simulink model "top_model"  (R2017a)
settings: Solver=ode23t  StartTime=0.0  StopTime=100  FixedStep=0.005  MaxStep=0.05  RelTol=1e-8  EnableMultiTasking=on
InitFcn:
  | load('DrivenData.mat');
  | load('vehicleParameters.mat');
undefined symbols (not defined in the file): B, C, CA, Cd, Cl, cogHeight, D, E, F, frontArea, frontBrakeBias, mass, maxBrakingTorque, maxPower, maxTorque, P, R, rearWeightDist, trackWidth, wheelBase
(part 1 of 2)
settings Model: Creator=The MathWorks, Inc.  LastModifiedBy=Jianming
settings SolverCC: MaxConsecutiveMinStep=5
settings DataIOCC: LimitDataPoints=on
settings OptimizationCC: LifeSpan=inf
settings DebuggingCC: AllowSymbolicDim=off  SFUnexpectedBacktrackingDiag=warning  SFNoUnconditionalDefaultTransitionDiag=warning  SFExecutionAtInitializationDiag=none
settings ModelReferenceCC: PropagateSignalLabelsOutOfModel=off
settings GRTTargetCC: TargetLangStandard=C89/C90 (ANSI)
settings ConfigComp: CovMetricSettings=dw  CovHtmlReporting=on  CovSaveCumulativeToWorkspaceVar=on  CovSaveSingleToWorkspaceVar=on  CovExternalEMLEnable=off

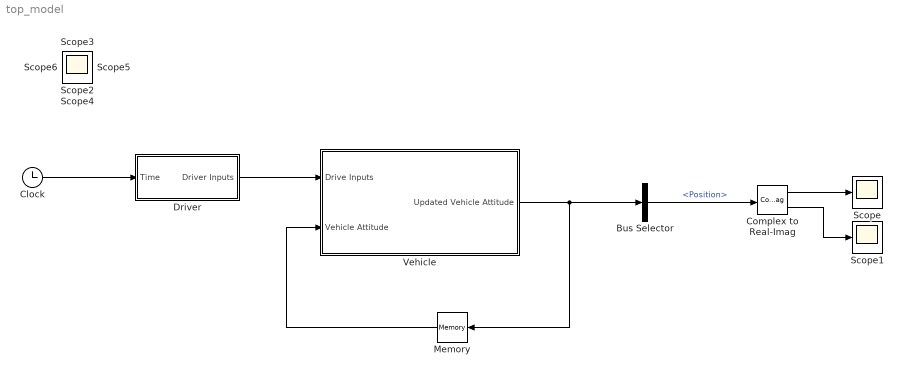
== system top_model ==
  Bus Selector : BusSelector  OutputSignals=Position
  Clock : Clock
  Complex to Real-Imag : ComplexToRealImag
  "Driver " : Subsystem
  Memory : Memory
  Scope{,1..6} (7 alike) : Scope
  Vehicle : Subsystem
  wires:
  Clock/1 -> "Driver "/1(Time)
  "Driver "/1(Driver Inputs) -> Vehicle/1(Drive Inputs)
  Vehicle/1(Updated Vehicle Attitude) -> Bus Selector/1, Memory/1
  Bus Selector/1 -> Complex to Real-Imag/1  "<Position>"
  Memory/1 -> Vehicle/2(Vehicle Attitude)
  Complex to Real-Imag/1 -> Scope/1
  Complex to Real-Imag/2 -> Scope1/1

== system top_model/Driver  ==
  Time : Inport
  Brake : Lookup_n-D  NumberOfTableDimensions=1  BreakpointsForDimension1=[0, 2, 2.1, 10]  Table=[0, 0, 0, 0]  InternalRulePriority=Speed  RndMeth=Simplest  InputSameDT=on
  Bus Creator : BusCreator  Inputs=3
  Steering : Lookup_n-D  NumberOfTableDimensions=1  BreakpointsForDimension1=[0, 2, 2.1, 100]  Table=[0, 0, 0.05, 0.05]  InternalRulePriority=Speed  RndMeth=Simplest  InputSameDT=on
  Throttle : Lookup_n-D  NumberOfTableDimensions=1  BreakpointsForDimension1=[0, 10]  Table=[0, 0]  InternalRulePriority=Speed  RndMeth=Simplest  InputSameDT=on
  Driver Inputs : Outport
  wires:
  Bus Creator/1 -> Driver Inputs/1
  Steering/1 -> Bus Creator/1  "Steering"
  Throttle/1 -> Bus Creator/2  "Throttle"
  Brake/1 -> Bus Creator/3  "Brake"
  Time/1 -> Brake/1, Throttle/1, Steering/1

== system top_model/Vehicle ==
  Drive Inputs : Inport
  Vehicle Attitude : Inport  Port=2
  Control Systems : Subsystem
  Net Forces : Subsystem
  Slip Ratio : Subsystem
  Suspension : Subsystem
  Updating Forces : Subsystem
  Wheel Velocities : Subsystem
  Wheels : Subsystem
  Updated Vehicle Attitude : Outport
  wires:
  Drive Inputs/1 -> Control Systems/1(Driver Inputs)
  Vehicle Attitude/1 -> Slip Ratio/3(Vehicle Attitude), Net Forces/4(Vehicle Attitude), Suspension/1(Vehicle Attitude), Wheel Velocities/1(Vehicle Attitude), Control Systems/2(Vehicle Attitude)
  Control Systems/3(Slip Angle) -> Wheels/1(Slip Angle)
  Suspension/1(Wheel Parameters) -> Wheels/3(Wheel Parameters)
  Wheels/1(Wheel Forces) -> Net Forces/3(Wheel Forces)
  Net Forces/2(Vehicle Moments) -> Updating Forces/2(Vehicle Moments)
  Updating Forces/1(Updated Vehicle Attitude) -> Updated Vehicle Attitude/1
  Net Forces/1(Vehicle Forces) -> Updating Forces/1(Vehicle Force)
  Control Systems/2(Wheel Direction) -> Slip Ratio/1(Wheel Direction), Net Forces/2(Wheel Direction)
  Wheel Velocities/1(Wheel Velocities) -> Slip Ratio/2(Wheel Velocities), Control Systems/3(Wheel Velocities)
  Slip Ratio/1(Slip Ratio) -> Updating Forces/4(Slip Ratio), Wheels/2(Slip Ratio)
  Control Systems/1(Wheel Torque) -> Net Forces/1(Wheel Torque)
  Net Forces/3(Wheel Moments) -> Updating Forces/3(Wheel Moments)

== system top_model/Vehicle/Control Systems ==
  Driver Inputs : Inport
  Vehicle Attitude : Inport  Port=2
  Wheel Velocities : Inport  Port=3
  Brakes and Drivetrain : Subsystem
  Bus Selector : BusSelector  OutputSignals=Throttle,Brake,Steering
  Bus Selector1 : BusSelector  OutputSignals=Velocity,Rotation
  Steering : Subsystem
  Wheel Torque : Outport
  Wheel Direction : Outport  Port=2
  Slip Angle : Outport  Port=3
  wires:
  Driver Inputs/1 -> Bus Selector/1
  Steering/2(Slip Angle) -> Slip Angle/1
  Bus Selector/3 -> Steering/1(Steering Input)  "<Steering>"
  Brakes and Drivetrain/1(Wheel Torque) -> Wheel Torque/1
  Bus Selector/1 -> Brakes and Drivetrain/1(Throttle)  "<Throttle>"
  Bus Selector/2 -> Brakes and Drivetrain/2(Brake)  "<Brake>"
  Steering/1(Wheel Direction) -> Wheel Direction/1
  Vehicle Attitude/1 -> Bus Selector1/1
  Bus Selector1/1 -> Brakes and Drivetrain/3(Velocity)  "<Velocity>"
  Bus Selector1/2 -> Steering/2(Vehicle Rotation)  "<Rotation>"
  Wheel Velocities/1 -> Steering/3(Wheel Velocities)

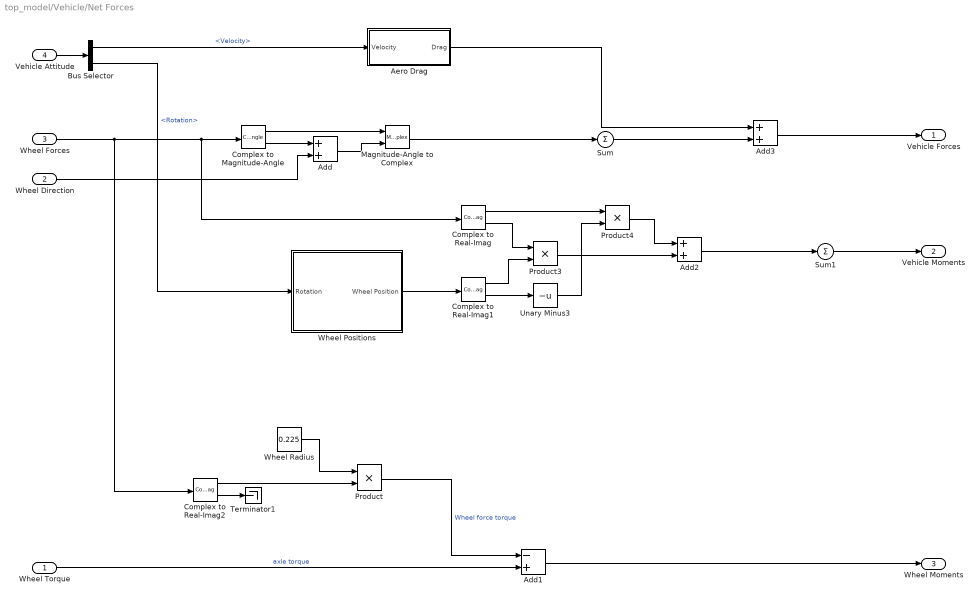
== system top_model/Vehicle/Net Forces ==
  Wheel Torque : Inport
  Wheel Direction : Inport  Port=2
  Wheel Forces : Inport  Port=3
  Vehicle Attitude : Inport  Port=4
  Add : Sum
  Add1 : Sum  Inputs=-+
  Add2 : Sum
  Add3 : Sum
  Aero Drag : Subsystem
  Bus Selector : BusSelector  OutputSignals=Velocity,Rotation
  Complex to Magnitude-Angle : ComplexToMagnitudeAngle
  Complex to Real-Imag : ComplexToRealImag
  Complex to Real-Imag1 : ComplexToRealImag
  Complex to Real-Imag2 : ComplexToRealImag
  Magnitude-Angle to Complex : MagnitudeAngleToComplex
  Product : Product
  Product3 : Product
  Product4 : Product
  Sum : Sum  Inputs=+
  Sum1 : Sum  Inputs=+
  Terminator1 : Terminator
  Unary Minus3 : UnaryMinus
  Wheel Positions : Subsystem
  Wheel Radius : Constant  Value=0.225
  Vehicle Forces : Outport
  Vehicle Moments : Outport  Port=2
  Wheel Moments : Outport  Port=3
  wires:
  Wheel Forces/1 -> Complex to Real-Imag/1, Complex to Magnitude-Angle/1, Complex to Real-Imag2/1
  Magnitude-Angle to Complex/1 -> Sum/1
  Complex to Magnitude-Angle/1 -> Magnitude-Angle to Complex/1
  Vehicle Attitude/1 -> Bus Selector/1
  Complex to Real-Imag/2 -> Product3/1
  Complex to Real-Imag1/1 -> Product3/2
  Complex to Real-Imag1/2 -> Unary Minus3/1
  Complex to Real-Imag/1 -> Product4/1
  Unary Minus3/1 -> Product4/2
  Product4/1 -> Add2/1
  Product3/1 -> Add2/2
  Bus Selector/1 -> Aero Drag/1(Velocity)  "<Velocity>"
  Sum/1 -> Add3/2
  Aero Drag/1(Drag) -> Add3/1
  Add3/1 -> Vehicle Forces/1
  Sum1/1 -> Vehicle Moments/1
  Add2/1 -> Sum1/1
  Complex to Magnitude-Angle/2 -> Add/1
  Wheel Direction/1 -> Add/2
  Add/1 -> Magnitude-Angle to Complex/2
  Complex to Real-Imag2/2 -> Terminator1/1
  Wheel Positions/1(Wheel Position) -> Complex to Real-Imag1/1
  Bus Selector/2 -> Wheel Positions/1(Rotation)  "<Rotation>"
  Wheel Torque/1 -> Add1/2  "axle torque"
  Product/1 -> Add1/1  "Wheel force torque"
  Add1/1 -> Wheel Moments/1
  Complex to Real-Imag2/1 -> Product/2
  Wheel Radius/1 -> Product/1

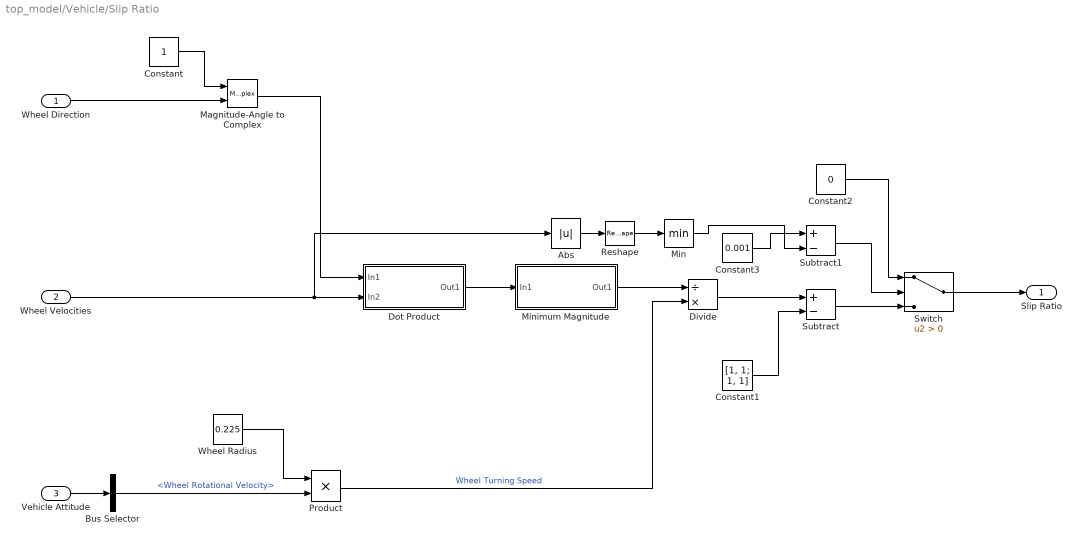
== system top_model/Vehicle/Slip Ratio ==
  Wheel Direction : Inport
  Wheel Velocities : Inport  Port=2
  Vehicle Attitude : Inport  Port=3
  Abs : Abs
  Bus Selector : BusSelector  OutputSignals=Wheel Rotational Velocity
  Constant : Constant
  Constant1 : Constant  Value=[1, 1; 1, 1]
  Constant2 : Constant  Value=0
  Constant3 : Constant  Value=0.001
  Divide : Product  Inputs=/*
  Dot Product : Subsystem
  Magnitude-Angle to Complex : MagnitudeAngleToComplex
  Min : MinMax
  Minimum Magnitude : Subsystem
  Product : Product
  Reshape : Reshape
  Subtract : Sum  Inputs=+-
  Subtract1 : Sum  Inputs=+-
  Switch : Switch  Criteria=u2 > Threshold
  Wheel Radius : Constant  Value=0.225
  Slip Ratio : Outport
  wires:
  Vehicle Attitude/1 -> Bus Selector/1
  Wheel Direction/1 -> Magnitude-Angle to Complex/2
  Constant/1 -> Magnitude-Angle to Complex/1
  Wheel Velocities/1 -> Abs/1, Dot Product/2(In2)
  Magnitude-Angle to Complex/1 -> Dot Product/1(In1)
  Dot Product/1(Out1) -> Minimum Magnitude/1(In1)
  Bus Selector/1 -> Product/2  "<Wheel Rotational Velocity>"
  Wheel Radius/1 -> Product/1
  Minimum Magnitude/1(Out1) -> Divide/1
  Product/1 -> Divide/2  "Wheel Turning Speed"
  Divide/1 -> Subtract/1
  Constant1/1 -> Subtract/2
  Subtract/1 -> Switch/3
  Subtract1/1 -> Switch/2
  Constant2/1 -> Switch/1
  Constant3/1 -> Subtract1/1
  Min/1 -> Subtract1/2
  Abs/1 -> Reshape/1
  Reshape/1 -> Min/1
  Switch/1 -> Slip Ratio/1

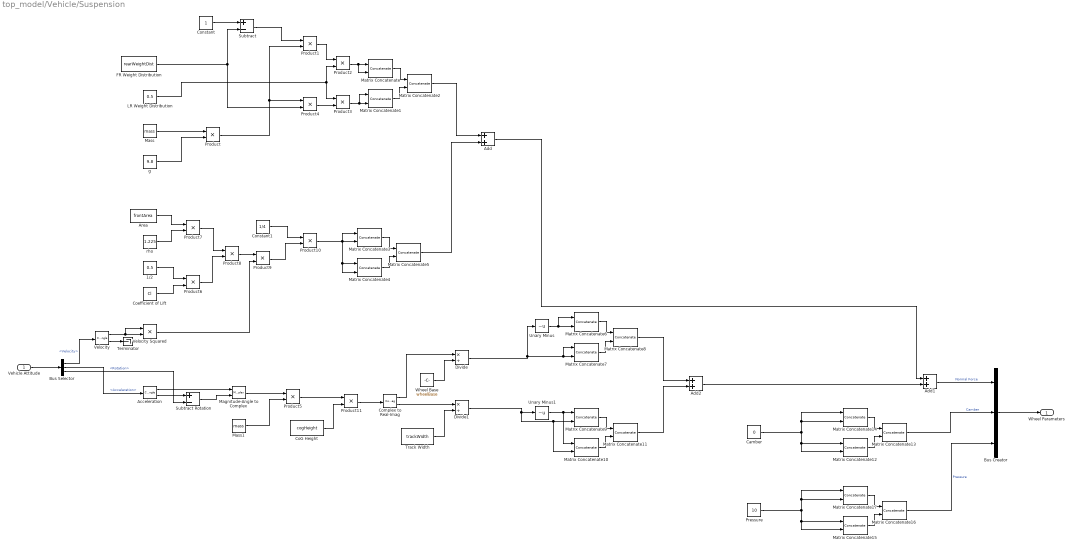
== system top_model/Vehicle/Suspension ==
  Vehicle Attitude : Inport
  1/2 : Constant  Value=0.5
  Acceleration : ComplexToMagnitudeAngle
  Add : Sum
  Add1 : Sum
  Add2 : Sum
  Area : Constant  Value=frontArea
  Bus Creator : BusCreator  Inputs=3
  Bus Selector : BusSelector  OutputSignals=Velocity,Acceleration,Rotation
  Camber : Constant  Value=0
  CoG Height : Constant  Value=cogHeight
  Coefficient of Lift : Constant  Value=Cl
  Complex to Real-Imag : ComplexToRealImag
  Constant : Constant
  Constant1 : Constant  Value=1/4
  Divide : Product  Inputs=*/
  Divide1 : Product  Inputs=*/
  FR Weight Distribution : Constant  Value=rearWeightDist
  LR Weight Distribution : Constant  Value=0.5
  Magnitude-Angle to Complex : MagnitudeAngleToComplex
  Mass : Constant  Value=mass
  Mass1 : Constant  Value=mass
  Matrix Concatenate{,1,3..4,6..7,9..10,12,14..15,17} (12 alike) : Concatenate  Mode=Multidimensional array  ConcatenateDimension=2
  Matrix Concatenate{2,5,8,11,13,16} (6 alike) : Concatenate  Mode=Multidimensional array
  Pressure : Constant  Value=10
  Product{,1..11} (12 alike) : Product
  Subtract : Sum  Inputs=+-
  Subtract Rotation : Sum  Inputs=+-
  Terminator : Terminator
  Track Width : Constant  Value=trackWidth
  Unary Minus : UnaryMinus
  Unary Minus1 : UnaryMinus
  Velocity : ComplexToMagnitudeAngle
  Velocity Squared : Product
  Wheel Base : Constant  Value=wheelBase
  g : Constant  Value=9.8
  rho : Constant  Value=1.225
  Wheel Parameters : Outport
  wires:
  Bus Creator/1 -> Wheel Parameters/1
  Mass/1 -> Product/1
  g/1 -> Product/2
  Constant/1 -> Subtract/1
  FR Weight Distribution/1 -> Product4/2, Subtract/2
  Matrix Concatenate/1 -> Matrix Concatenate2/1
  Matrix Concatenate1/1 -> Matrix Concatenate2/2
  Subtract/1 -> Product1/1
  Product/1 -> Product4/1, Product1/2
  Product1/1 -> Product2/1
  LR Weight Distribution/1 -> Product3/1, Product2/2
  Product2/1 -> Matrix Concatenate/2, Matrix Concatenate/1
  Product3/1 -> Matrix Concatenate1/1, Matrix Concatenate1/2
  Product4/1 -> Product3/2
  Area/1 -> Product7/1
  rho/1 -> Product7/2
  1/2/1 -> Product6/1
  Coefficient of Lift/1 -> Product6/2
  Product7/1 -> Product8/1
  Product6/1 -> Product8/2
  Product8/1 -> Product9/1
  Velocity Squared/1 -> Product9/2
  Constant1/1 -> Product10/1
  Product9/1 -> Product10/2
  Matrix Concatenate3/1 -> Matrix Concatenate5/1
  Matrix Concatenate4/1 -> Matrix Concatenate5/2
  Product10/1 -> Matrix Concatenate4/2, Matrix Concatenate4/1, Matrix Concatenate3/1, Matrix Concatenate3/2
  Matrix Concatenate2/1 -> Add/1
  Matrix Concatenate5/1 -> Add/2
  Add1/1 -> Bus Creator/1  "Normal Force"
  Add/1 -> Add1/1
  Velocity/1 -> Velocity Squared/1, Velocity Squared/2
  Velocity/2 -> Terminator/1
  Acceleration/1 -> Magnitude-Angle to Complex/1
  Acceleration/2 -> Subtract Rotation/1
  Subtract Rotation/1 -> Magnitude-Angle to Complex/2
  Magnitude-Angle to Complex/1 -> Product5/1
  Mass1/1 -> Product5/2
  Product5/1 -> Product11/1
  CoG Height/1 -> Product11/2
  Product11/1 -> Complex to Real-Imag/1
  Complex to Real-Imag/1 -> Divide/1
  Wheel Base/1 -> Divide/2
  Complex to Real-Imag/2 -> Divide1/1
  Track Width/1 -> Divide1/2
  Matrix Concatenate7/1 -> Matrix Concatenate8/2
  Matrix Concatenate6/1 -> Matrix Concatenate8/1
  Divide/1 -> Matrix Concatenate7/1, Matrix Concatenate7/2, Unary Minus/1
  Matrix Concatenate9/1 -> Matrix Concatenate11/1
  Matrix Concatenate10/1 -> Matrix Concatenate11/2
  Matrix Concatenate8/1 -> Add2/1
  Matrix Concatenate11/1 -> Add2/2
  Add2/1 -> Add1/2
  Matrix Concatenate14/1 -> Matrix Concatenate13/1
  Matrix Concatenate12/1 -> Matrix Concatenate13/2
  Matrix Concatenate17/1 -> Matrix Concatenate16/1
  Matrix Concatenate15/1 -> Matrix Concatenate16/2
  Matrix Concatenate13/1 -> Bus Creator/2  "Camber"
  Matrix Concatenate16/1 -> Bus Creator/3  "Pressure"
  Camber/1 -> Matrix Concatenate12/1, Matrix Concatenate12/2, Matrix Concatenate14/2, Matrix Concatenate14/1
  Pressure/1 -> Matrix Concatenate15/2, Matrix Concatenate15/1, Matrix Concatenate17/2, Matrix Concatenate17/1
  Vehicle Attitude/1 -> Bus Selector/1
  Bus Selector/1 -> Velocity/1  "<Velocity>"
  Bus Selector/2 -> Acceleration/1  "<Acceleration>"
  Bus Selector/3 -> Subtract Rotation/2  "<Rotation>"
  Unary Minus/1 -> Matrix Concatenate6/1, Matrix Concatenate6/2
  Divide1/1 -> Unary Minus1/1, Matrix Concatenate10/2, Matrix Concatenate9/2
  Unary Minus1/1 -> Matrix Concatenate10/1, Matrix Concatenate9/1

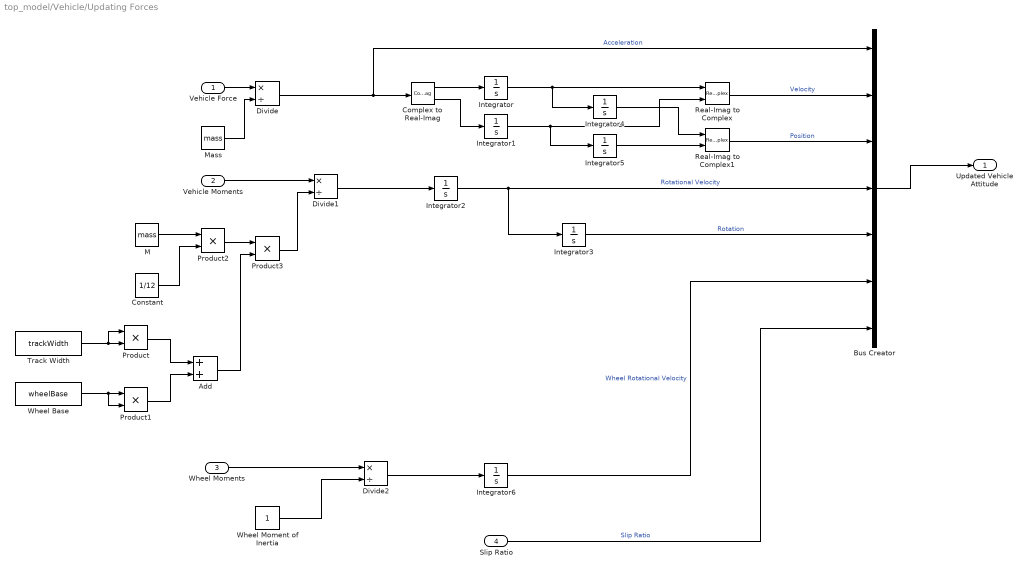
== system top_model/Vehicle/Updating Forces ==
  Vehicle Force : Inport
  Vehicle Moments : Inport  Port=2
  Wheel Moments : Inport  Port=3
  Slip Ratio : Inport  Port=4
  Add : Sum
  Bus Creator : BusCreator  Inputs=7
  Complex to Real-Imag : ComplexToRealImag
  Constant : Constant  Value=1/12
  Divide : Product  Inputs=*/
  Divide1 : Product  Inputs=*/
  Divide2 : Product  Inputs=*/
  Integrator : Integrator  InitialCondition=10
  Integrator{1..5} (5 alike) : Integrator
  Integrator6 : Integrator  InitialCondition=[0, 0; 0, 0]
  M : Constant  Value=mass
  Mass : Constant  Value=mass
  Product{,1..3} (4 alike) : Product
  Real-Imag to Complex : RealImagToComplex
  Real-Imag to Complex1 : RealImagToComplex
  Track Width : Constant  Value=trackWidth
  Wheel Base : Constant  Value=wheelBase
  Wheel Moment of Inertia : Constant
  Updated Vehicle Attitude : Outport
  wires:
  Divide/1 -> Complex to Real-Imag/1, Bus Creator/1  "Acceleration"
  Real-Imag to Complex/1 -> Bus Creator/2  "Velocity"
  Real-Imag to Complex1/1 -> Bus Creator/3  "Position"
  Integrator3/1 -> Bus Creator/5  "Rotation"
  Integrator2/1 -> Integrator3/1, Bus Creator/4  "Rotational Velocity"
  Bus Creator/1 -> Updated Vehicle Attitude/1
  Complex to Real-Imag/1 -> Integrator/1
  Complex to Real-Imag/2 -> Integrator1/1
  Integrator/1 -> Real-Imag to Complex/1, Integrator4/1
  Integrator1/1 -> Integrator5/1, Real-Imag to Complex/2
  Integrator5/1 -> Real-Imag to Complex1/2
  Integrator4/1 -> Real-Imag to Complex1/1
  Vehicle Force/1 -> Divide/1
  Mass/1 -> Divide/2
  Divide1/1 -> Integrator2/1
  Vehicle Moments/1 -> Divide1/1
  Track Width/1 -> Product/1, Product/2
  Wheel Base/1 -> Product1/2, Product1/1
  Product/1 -> Add/1
  Product1/1 -> Add/2
  M/1 -> Product2/1
  Constant/1 -> Product2/2
  Product2/1 -> Product3/1
  Add/1 -> Product3/2
  Product3/1 -> Divide1/2
  Wheel Moments/1 -> Divide2/1
  Wheel Moment of Inertia/1 -> Divide2/2
  Divide2/1 -> Integrator6/1
  Integrator6/1 -> Bus Creator/6  "Wheel Rotational Velocity"
  Slip Ratio/1 -> Bus Creator/7  "Slip Ratio"

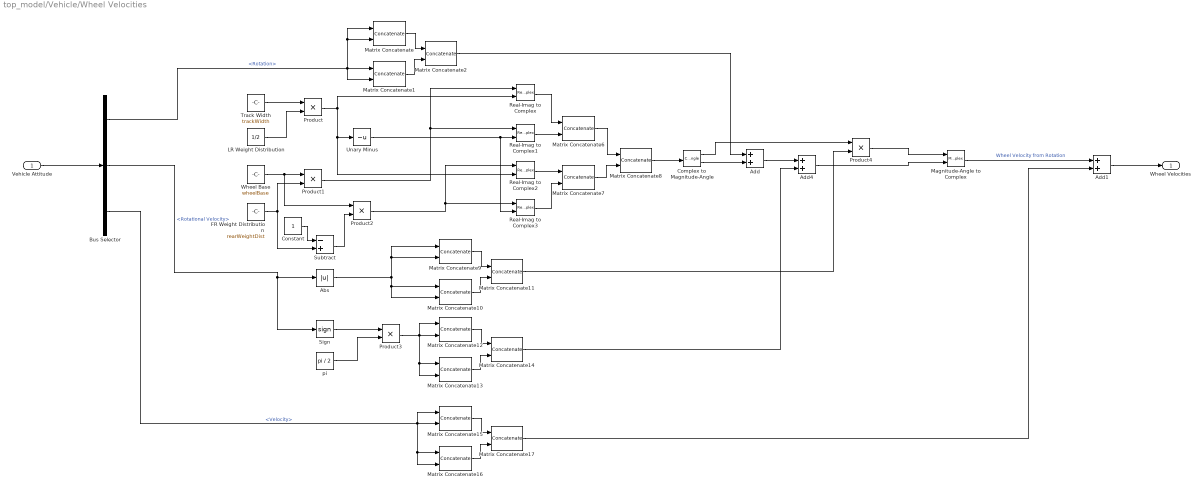
== system top_model/Vehicle/Wheel Velocities ==
  Vehicle Attitude : Inport
  Abs : Abs
  Add : Sum
  Add1 : Sum
  Add4 : Sum
  Bus Selector : BusSelector  OutputSignals=Rotation,Rotational Velocity,Velocity
  Complex to Magnitude-Angle : ComplexToMagnitudeAngle
  Constant : Constant
  FR Weight Distribution : Constant  Value=rearWeightDist
  LR Weight Distribution : Constant  Value=1/2
  Magnitude-Angle to Complex : MagnitudeAngleToComplex
  Matrix Concatenate{,1,6..7,9..10,12..13,15..16} (10 alike) : Concatenate  Mode=Multidimensional array  ConcatenateDimension=2
  Matrix Concatenate{2,8,11,14,17} (5 alike) : Concatenate  Mode=Multidimensional array
  Product{,1..4} (5 alike) : Product
  Real-Imag to Complex{,1..3} (4 alike) : RealImagToComplex
  Sign : Signum
  Subtract : Sum  Inputs=-+
  Track Width : Constant  Value=trackWidth
  Unary Minus : UnaryMinus
  Wheel Base : Constant  Value=wheelBase
  pi : Constant  Value=pi / 2
  Wheel Velocities : Outport
  wires:
  Matrix Concatenate6/1 -> Matrix Concatenate8/1
  Product3/1 -> Matrix Concatenate13/2, Matrix Concatenate13/1, Matrix Concatenate12/1, Matrix Concatenate12/2
  Matrix Concatenate11/1 -> Product4/2
  Wheel Base/1 -> Product2/1, Product1/1
  Matrix Concatenate14/1 -> Add4/2
  LR Weight Distribution/1 -> Product/2
  Real-Imag to Complex1/1 -> Matrix Concatenate6/2
  Real-Imag to Complex3/1 -> Matrix Concatenate7/2
  Matrix Concatenate8/1 -> Complex to Magnitude-Angle/1
  Product4/1 -> Magnitude-Angle to Complex/1
  Real-Imag to Complex/1 -> Matrix Concatenate6/1
  pi/1 -> Product3/2
  Bus Selector/1 -> Matrix Concatenate1/2, Matrix Concatenate/2, Matrix Concatenate/1, Matrix Concatenate1/1  "<Rotation>"
  Matrix Concatenate13/1 -> Matrix Concatenate14/2
  Matrix Concatenate9/1 -> Matrix Concatenate11/1
  Matrix Concatenate10/1 -> Matrix Concatenate11/2
  Real-Imag to Complex2/1 -> Matrix Concatenate7/1
  Add/1 -> Add4/1
  Product/1 -> Real-Imag to Complex/2, Real-Imag to Complex2/2, Unary Minus/1
  Track Width/1 -> Product/1
  Product2/1 -> Real-Imag to Complex3/1, Real-Imag to Complex2/1
  Bus Selector/2 -> Sign/1, Abs/1  "<Rotational Velocity>"
  Constant/1 -> Subtract/1
  Complex to Magnitude-Angle/2 -> Add/2
  Sign/1 -> Product3/1
  Matrix Concatenate7/1 -> Matrix Concatenate8/2
  Unary Minus/1 -> Real-Imag to Complex3/2, Real-Imag to Complex1/2
  Product1/1 -> Real-Imag to Complex1/1, Real-Imag to Complex/1
  Add4/1 -> Magnitude-Angle to Complex/2
  Complex to Magnitude-Angle/1 -> Product4/1
  Matrix Concatenate1/1 -> Matrix Concatenate2/2
  FR Weight Distribution/1 -> Subtract/2, Product1/2
  Matrix Concatenate2/1 -> Add/1
  Matrix Concatenate12/1 -> Matrix Concatenate14/1
  Subtract/1 -> Product2/2
  Magnitude-Angle to Complex/1 -> Add1/1  "Wheel Velocity from Rotation"
  Abs/1 -> Matrix Concatenate10/2, Matrix Concatenate10/1, Matrix Concatenate9/2, Matrix Concatenate9/1
  Vehicle Attitude/1 -> Bus Selector/1
  Bus Selector/3 -> Matrix Concatenate16/2, Matrix Concatenate16/1, Matrix Concatenate15/1, Matrix Concatenate15/2  "<Velocity>"
  Matrix Concatenate16/1 -> Matrix Concatenate17/2
  Matrix Concatenate17/1 -> Add1/2
  Matrix Concatenate15/1 -> Matrix Concatenate17/1
  Add1/1 -> Wheel Velocities/1
  Matrix Concatenate/1 -> Matrix Concatenate2/1

== system top_model/Vehicle/Wheels ==
  Slip Angle : Inport
  Slip Ratio : Inport  Port=2
  Wheel Parameters : Inport  Port=3
  Tire Forces : Subsystem
  Wheel Forces : Outport
  wires:
  Slip Angle/1 -> Tire Forces/1(Slip Angle)
  Wheel Parameters/1 -> Tire Forces/3(Wheel Parameters)
  Tire Forces/1(Wheel Forces) -> Wheel Forces/1
  Slip Ratio/1 -> Tire Forces/2(Slip Ratio)

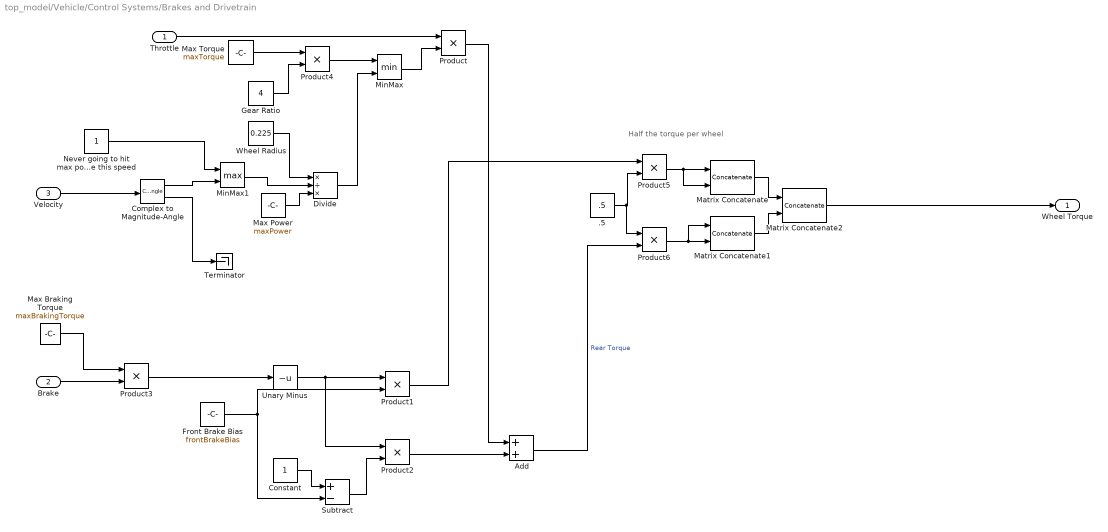
== system top_model/Vehicle/Control Systems/Brakes and Drivetrain ==
  note: Half the torque per wheel
  Throttle : Inport
  Brake : Inport  Port=2
  Velocity : Inport  Port=3
  .5 : Constant  Value=.5
  Add : Sum
  Complex to Magnitude-Angle : ComplexToMagnitudeAngle
  Constant : Constant
  Divide : Product  Inputs=*/*
  Front Brake Bias : Constant  Value=frontBrakeBias
  Gear Ratio : Constant  Value=4
  Matrix Concatenate : Concatenate  Mode=Multidimensional array  ConcatenateDimension=2
  Matrix Concatenate1 : Concatenate  Mode=Multidimensional array  ConcatenateDimension=2
  Matrix Concatenate2 : Concatenate  Mode=Multidimensional array
  Max Braking Torque : Constant  Value=maxBrakingTorque
  Max Power : Constant  Value=maxPower
  Max Torque : Constant  Value=maxTorque
  MinMax : MinMax  Inputs=2
  MinMax1 : MinMax  Function=max  Inputs=2
  Never going to hit max power before this speed : Constant
  Product{,1..6} (7 alike) : Product
  Subtract : Sum  Inputs=+-
  Terminator : Terminator
  Unary Minus : UnaryMinus
  Wheel Radius : Constant  Value=0.225
  Wheel Torque : Outport
  wires:
  Throttle/1 -> Product/1
  Front Brake Bias/1 -> Subtract/2, Product1/2
  Constant/1 -> Subtract/1
  Subtract/1 -> Product2/2
  Brake/1 -> Product3/2
  Unary Minus/1 -> Product2/1, Product1/1
  Max Braking Torque/1 -> Product3/1
  Product2/1 -> Add/2
  Product/1 -> Add/1
  Matrix Concatenate/1 -> Matrix Concatenate2/1
  Matrix Concatenate1/1 -> Matrix Concatenate2/2
  Matrix Concatenate2/1 -> Wheel Torque/1
  Max Power/1 -> Divide/3
  MinMax/1 -> Product/2
  Divide/1 -> MinMax/2
  Wheel Radius/1 -> Divide/1
  Complex to Magnitude-Angle/2 -> Terminator/1
  Velocity/1 -> Complex to Magnitude-Angle/1
  MinMax1/1 -> Divide/2
  Complex to Magnitude-Angle/1 -> MinMax1/2
  Never going to hit max power before this speed/1 -> MinMax1/1
  Product3/1 -> Unary Minus/1
  Max Torque/1 -> Product4/1
  Product4/1 -> MinMax/1
  Gear Ratio/1 -> Product4/2
  Product6/1 -> Matrix Concatenate1/2, Matrix Concatenate1/1
  Product5/1 -> Matrix Concatenate/2, Matrix Concatenate/1
  .5/1 -> Product6/1, Product5/2
  Add/1 -> Product6/2  "Rear Torque"
  Product1/1 -> Product5/1

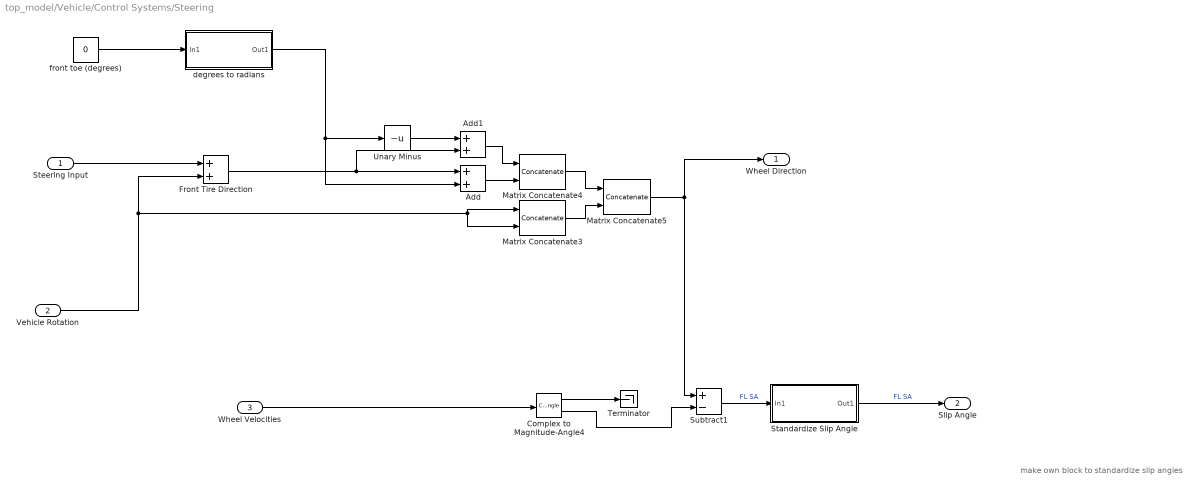
== system top_model/Vehicle/Control Systems/Steering ==
  note: make own block to standardize slip angles
  Steering Input : Inport
  Vehicle Rotation : Inport  Port=2
  Wheel Velocities : Inport  Port=3
  Add : Sum
  Add1 : Sum
  Complex to Magnitude-Angle4 : ComplexToMagnitudeAngle
  Front Tire Direction : Sum
  Matrix Concatenate3 : Concatenate  Mode=Multidimensional array  ConcatenateDimension=2
  Matrix Concatenate4 : Concatenate  Mode=Multidimensional array  ConcatenateDimension=2
  Matrix Concatenate5 : Concatenate  Mode=Multidimensional array
  Standardize Slip Angle : Subsystem
  Subtract1 : Sum  Inputs=+-
  Terminator : Terminator
  Unary Minus : UnaryMinus
  degrees to radians : Subsystem
  front toe (degrees) : Constant  Value=0
  Wheel Direction : Outport
  Slip Angle : Outport  Port=2
  wires:
  Steering Input/1 -> Front Tire Direction/1
  Complex to Magnitude-Angle4/1 -> Terminator/1
  Complex to Magnitude-Angle4/2 -> Subtract1/2
  Vehicle Rotation/1 -> Matrix Concatenate3/2, Matrix Concatenate3/1, Front Tire Direction/2
  Matrix Concatenate4/1 -> Matrix Concatenate5/1
  Matrix Concatenate3/1 -> Matrix Concatenate5/2
  Matrix Concatenate5/1 -> Wheel Direction/1, Subtract1/1
  Standardize Slip Angle/1(Out1) -> Slip Angle/1  "FL SA"
  Wheel Velocities/1 -> Complex to Magnitude-Angle4/1
  front toe (degrees)/1 -> degrees to radians/1(In1)
  Add/1 -> Matrix Concatenate4/2
  Front Tire Direction/1 -> Add1/2, Add/1
  degrees to radians/1(Out1) -> Unary Minus/1, Add/2
  Add1/1 -> Matrix Concatenate4/1
  Unary Minus/1 -> Add1/1
  Subtract1/1 -> Standardize Slip Angle/1(In1)  "FL SA"

== system top_model/Vehicle/Net Forces/Aero Drag ==
  Velocity : Inport
  1/2 : Constant  Value=-0.5
  Area : Constant  Value=frontArea
  Coefficient of Drag : Constant  Value=Cd
  Complex to Magnitude-Angle2 : ComplexToMagnitudeAngle
  Product{5..9} (5 alike) : Product
  Terminator : Terminator
  rho : Constant  Value=1.225
  Drag : Outport
  wires:
  Product7/1 -> Product9/2
  Product8/1 -> Product9/1
  Coefficient of Drag/1 -> Product7/2
  Product9/1 -> Product6/1
  Complex to Magnitude-Angle2/1 -> Product5/2
  1/2/1 -> Product7/1
  Complex to Magnitude-Angle2/2 -> Terminator/1
  rho/1 -> Product8/2
  Product5/1 -> Product6/2
  Area/1 -> Product8/1
  Velocity/1 -> Complex to Magnitude-Angle2/1, Product5/1
  Product6/1 -> Drag/1

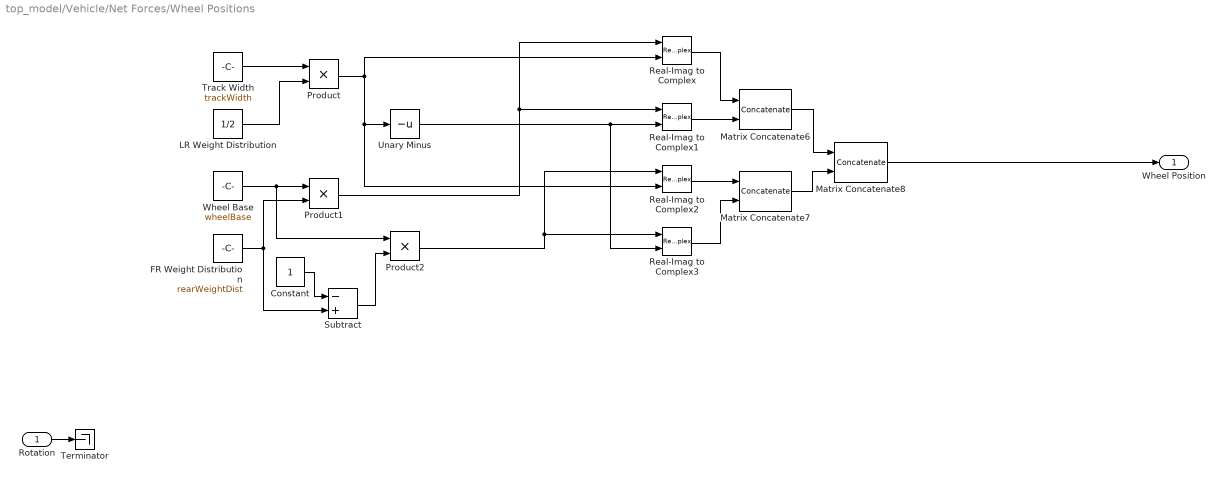
== system top_model/Vehicle/Net Forces/Wheel Positions ==
  Rotation : Inport
  Constant : Constant
  FR Weight Distribution : Constant  Value=rearWeightDist
  LR Weight Distribution : Constant  Value=1/2
  Matrix Concatenate6 : Concatenate  Mode=Multidimensional array  ConcatenateDimension=2
  Matrix Concatenate7 : Concatenate  Mode=Multidimensional array  ConcatenateDimension=2
  Matrix Concatenate8 : Concatenate  Mode=Multidimensional array
  Product : Product
  Product1 : Product
  Product2 : Product
  Real-Imag to Complex{,1..3} (4 alike) : RealImagToComplex
  Subtract : Sum  Inputs=-+
  Terminator : Terminator
  Track Width : Constant  Value=trackWidth
  Unary Minus : UnaryMinus
  Wheel Base : Constant  Value=wheelBase
  Wheel Position : Outport
  wires:
  Subtract/1 -> Product2/2
  Real-Imag to Complex2/1 -> Matrix Concatenate7/1
  Product1/1 -> Real-Imag to Complex1/1, Real-Imag to Complex/1
  Constant/1 -> Subtract/1
  Real-Imag to Complex3/1 -> Matrix Concatenate7/2
  Wheel Base/1 -> Product2/1, Product1/1
  Unary Minus/1 -> Real-Imag to Complex3/2, Real-Imag to Complex1/2
  Track Width/1 -> Product/1
  FR Weight Distribution/1 -> Subtract/2, Product1/2
  Matrix Concatenate8/1 -> Wheel Position/1
  LR Weight Distribution/1 -> Product/2
  Product/1 -> Real-Imag to Complex/2, Real-Imag to Complex2/2, Unary Minus/1
  Matrix Concatenate6/1 -> Matrix Concatenate8/1
  Matrix Concatenate7/1 -> Matrix Concatenate8/2
  Real-Imag to Complex1/1 -> Matrix Concatenate6/2
  Product2/1 -> Real-Imag to Complex3/1, Real-Imag to Complex2/1
  Real-Imag to Complex/1 -> Matrix Concatenate6/1
  Rotation/1 -> Terminator/1

== system top_model/Vehicle/Slip Ratio/Dot Product ==
  In1 : Inport
  In2 : Inport  Port=2
  Add : Sum
  Complex to Real-Imag : ComplexToRealImag
  Complex to Real-Imag1 : ComplexToRealImag
  Product : Product
  Product1 : Product
  Out1 : Outport
  wires:
  In1/1 -> Complex to Real-Imag/1
  In2/1 -> Complex to Real-Imag1/1
  Complex to Real-Imag/1 -> Product/1
  Complex to Real-Imag1/1 -> Product/2
  Complex to Real-Imag1/2 -> Product1/2
  Complex to Real-Imag/2 -> Product1/1
  Product/1 -> Add/1
  Product1/1 -> Add/2
  Add/1 -> Out1/1

== system top_model/Vehicle/Slip Ratio/Minimum Magnitude ==
  In1 : Inport
  0.001 m/s : Constant  Value=0.001 * [1, 1; 1, 1]
  Abs : Abs
  Constant : Constant
  Max : MinMax  Function=max  Inputs=2
  Product : Product
  Sign : Signum
  Switch : Switch  Criteria=u2 ~= 0
  Out1 : Outport
  wires:
  In1/1 -> Sign/1, Abs/1
  Abs/1 -> Max/2
  0.001 m/s/1 -> Max/1
  Max/1 -> Product/1
  Product/1 -> Out1/1
  Sign/1 -> Switch/2, Switch/1
  Constant/1 -> Switch/3
  Switch/1 -> Product/2

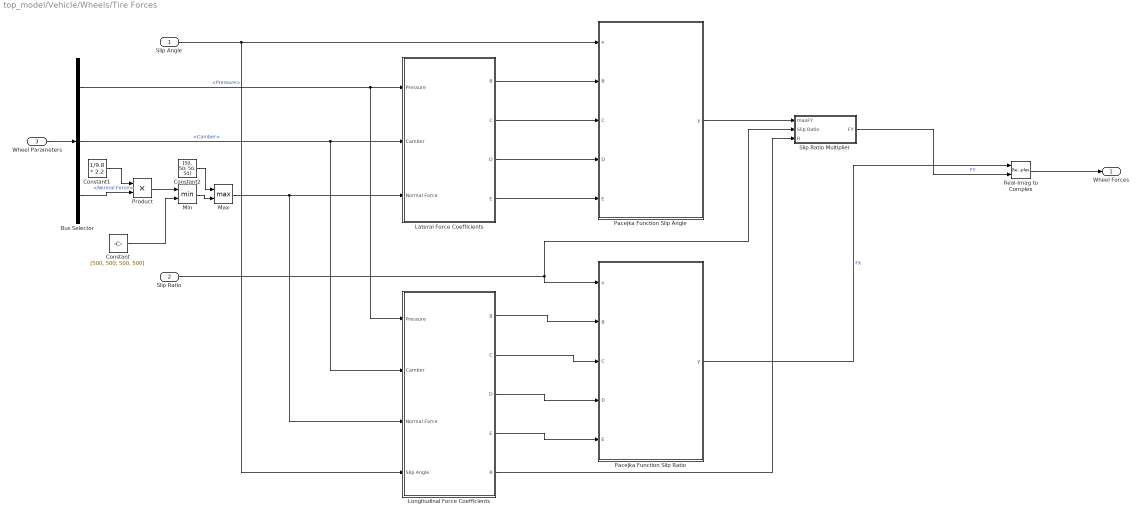
== system top_model/Vehicle/Wheels/Tire Forces ==
  Slip Angle : Inport
  Slip Ratio : Inport  Port=2
  Wheel Parameters : Inport  Port=3
  Bus Selector : BusSelector  OutputSignals=Pressure,Camber,Normal Force
  Constant : Constant  Value=[500, 500; 500, 500]
  Constant1 : Constant  Value=1/9.8 * 2.2
  Constant2 : Constant  Value=[50, 50; 50, 50]
  Lateral Force Coefficients : Subsystem  TreatAsAtomicUnit=on
  Longitudinal Force Coefficients : Subsystem  TreatAsAtomicUnit=on
  Max : MinMax  Function=max  Inputs=2
  Min : MinMax  Inputs=2
  Pacejka Function Slip Angle : Subsystem  TreatAsAtomicUnit=on
  Pacejka Function Slip Ratio : Subsystem  TreatAsAtomicUnit=on
  Product : Product
  Real-Imag to Complex : RealImagToComplex
  Slip Ratio Multiplier : Subsystem
  Wheel Forces : Outport
  wires:
  Bus Selector/1 -> Longitudinal Force Coefficients/1(Pressure), Lateral Force Coefficients/1(Pressure)  "<Pressure>"
  Lateral Force Coefficients/4(E) -> Pacejka Function Slip Angle/5(E)
  Longitudinal Force Coefficients/3(D) -> Pacejka Function Slip Ratio/4(D)
  Slip Ratio/1 -> Slip Ratio Multiplier/2(Slip Ratio), Pacejka Function Slip Ratio/1(x)
  Longitudinal Force Coefficients/2(C) -> Pacejka Function Slip Ratio/3(C)
  Lateral Force Coefficients/3(D) -> Pacejka Function Slip Angle/4(D)
  Lateral Force Coefficients/1(B) -> Pacejka Function Slip Angle/2("B ")
  Bus Selector/2 -> Longitudinal Force Coefficients/2(Camber), Lateral Force Coefficients/2(Camber)  "<Camber>"
  Lateral Force Coefficients/2(C) -> Pacejka Function Slip Angle/3(C)
  Longitudinal Force Coefficients/1(B) -> Pacejka Function Slip Ratio/2("B ")
  Longitudinal Force Coefficients/5(R) -> Slip Ratio Multiplier/3(R)
  Pacejka Function Slip Angle/1(y) -> Slip Ratio Multiplier/1(maxFY)
  Longitudinal Force Coefficients/4(E) -> Pacejka Function Slip Ratio/5(E)
  Slip Angle/1 -> Longitudinal Force Coefficients/4(Slip Angle), Pacejka Function Slip Angle/1(x)
  Slip Ratio Multiplier/1(FY) -> Real-Imag to Complex/2  "FY"
  Max/1 -> Longitudinal Force Coefficients/3(Normal Force), Lateral Force Coefficients/3(Normal Force)
  Pacejka Function Slip Ratio/1(y) -> Real-Imag to Complex/1  "FX"
  Wheel Parameters/1 -> Bus Selector/1
  Real-Imag to Complex/1 -> Wheel Forces/1
  Product/1 -> Min/1
  Bus Selector/3 -> Product/2  "<Normal Force>"
  Constant/1 -> Min/2
  Constant1/1 -> Product/1
  Min/1 -> Max/2
  Constant2/1 -> Max/1

== system top_model/Vehicle/Control Systems/Steering/Standardize Slip Angle ==
  In1 : Inport
  Constant : Constant  Value=2*pi
  Divide : Product  Inputs=*/
  Floor : Rounding  Operator=round
  Product : Product
  Subtract : Sum  Inputs=+-
  Out1 : Outport
  wires:
  In1/1 -> Divide/1
  Constant/1 -> Product/2, Divide/2
  Divide/1 -> Floor/1, Subtract/1
  Floor/1 -> Subtract/2
  Subtract/1 -> Product/1
  Product/1 -> Out1/1

== system top_model/Vehicle/Control Systems/Steering/degrees to radians ==
  In1 : Inport
  Constant : Constant  Value=pi
  Constant1 : Constant  Value=180
  Divide : Product  Inputs=*/
  Product : Product
  Out1 : Outport
  wires:
  In1/1 -> Product/1
  Divide/1 -> Product/2
  Constant/1 -> Divide/1
  Constant1/1 -> Divide/2
  Product/1 -> Out1/1

== system top_model/Vehicle/Wheels/Tire Forces/Lateral Force Coefficients ==
  Pressure : Inport
  Camber : Inport  Port=2
  Normal Force : Inport  Port=3
  B Coeff Lookup : Lookup_n-D  NumberOfTableDimensions=3  BreakpointsForDimension1=[8, 10, 12, 14]  BreakpointsForDimension2=[0, 1, 2, 3, 4]  BreakpointsForDimension3=[50, 100, 150, 200, 250]  Table=|  ExtrapMethod=Clip  UseLastTableValue=on  InternalRulePriority=Speed  OutDataTypeStr=double  RndMeth=Simplest  InputSameDT=on
      | reshape([  20.818832404187567
      | 
      |   14.367494448641477
      | 
      |   12.274690678601786
      | 
      |   11.293912922988415
      | 
      |    7.367396095983257
      | 
      |   19.210891617304256
      | 
      |   12.840234737487171
      | 
      |   12.496762621621839
      | 
      |   11.453772890679275
      | 
      |   15.012989677811818
      | 
      |   18.116205640570389
      | 
      |   12.694930618722518
      | 
      |   12.993552675343423
      | 
      |   12.768698690676276
      | 
      |   15.597027649583856
      | 
      |   17.099072313079052
      | 
      |   14.766202413755879
      | 
      |   13.327554423191769
      | 
      |   13.063311213885155
      | 
      |   15.910883809889334
      | 
      |   14.207900238745053
      | 
      |   13.765868089842158
      | 
      |   13.052548163652569
      | 
      |   13.338566818030792
      | 
      |   15.695567754732826
      | 
      |   23.732773081907823
      | 
      |   16.997636621348992
      | 
      |   11.613155614765923
      | 
      |    9.532866955373180
      | 
      |    9.010728172538675
      | 
      |   22.836417594446576
      | 
      |   16.296773960426442
      | 
      |   11.510860173007547
      | 
      |    8.184958764009460
      | 
      |    9.761841733187952
      | 
      |   24.934500317170905
      | 
      |   15.099908624820570
      | 
      |   10.976805066702900
      | 
      |   10.570404520571014
      | 
      |   10.728649625188515
      | 
      |   21.474620744593143
      | 
      |   13.419195849270638
      | 
      |   10.373984287779795
      | 
      |   11.554254710092200
      | 
      |   11.346007133003370
      | 
      |   17.322218391087770
      | 
      |   11.442857626569422
      | 
      |   10.556252190723793
      | 
      |   12.164583456050584
      | 
      |   11.699361362114816
      | 
      |   25.336272773839713
      | 
      |   18.282094133734876
      | 
      |   13.368403511904145
      | 
      |    9.545313579052614
      | 
      |    7.719908946702572
      | 
      |   24.663898162299354
      | 
      |   17.574326572836295
      | 
      |   13.290583804340905
      | 
      |    9.945940758183967
      | 
      |    8.021667377316069
      | 
      |   23.551837396212719
      | 
      |   17.894415503234320
      | 
      |   12.589121175788685
      | 
      |    9.884076462450226
      | 
      |    8.089858652786313
      | 
      |   24.164202006116497
      | 
      |   15.450581284070417
      | 
      |   12.159804191524803
      | 
      |    9.851909920187639
      | 
      |    7.985382615809471
      | 
      |   23.762666406252247
      | 
      |   13.017363999235569
      | 
      |   10.772936855538736
      | 
      |   12.159186218944935
      | 
      |   11.818329663411943
      | 
      |   22.489025207278520
      | 
      |   18.382753381379192
      | 
      |   13.703923768066133
      | 
      |    9.997112986808878
      | 
      |    8.609543337116151
      | 
      |   21.046279516590616
      | 
      |   17.584891301522227
      | 
      |   13.901154543649730
      | 
      |   10.548269205960951
      | 
      |    8.606547290854801
      | 
      |   21.928568285109048
      | 
      |   17.828157734724957
      | 
      |   13.293463133092075
      | 
      |   10.532385949033966
      | 
      |    8.772840965703812
      | 
      |   19.324191931659087
      | 
      |   15.908794115544467
      | 
      |   12.245294529149103
      | 
      |   10.241879291517760
      | 
      |    8.660574917528058
      | 
      |   24.450396050208408
      | 
      |   14.731074750848038
      | 
      |   11.439407920802067
      | 
      |   11.486704957172245
      | 
      |   11.834019695365980], [4 5 5])
  C Coeff Lookup : Lookup_n-D  NumberOfTableDimensions=3  BreakpointsForDimension1=[8 10 12 14]  BreakpointsForDimension2=[0 1 2 3 4]  BreakpointsForDimension3=[50 100 150 200 250]  Table=|  ExtrapMethod=Clip  UseLastTableValue=on  InternalRulePriority=Speed  RndMeth=Simplest  InputSameDT=on
      | reshape([   1.395907415451345
      | 
      |    1.515758093867311
      | 
      |    1.409721710254408
      | 
      |    1.228039178894097
      | 
      |    1.720229661265224
      | 
      |    1.414487346952960
      | 
      |    1.648635820365763
      | 
      |    1.375129632389121
      | 
      |    1.227132229080082
      | 
      |    0.462888890239916
      | 
      |    1.396003366270241
      | 
      |    1.626246598590263
      | 
      |    1.342950008179124
      | 
      |    1.077925909777369
      | 
      |    0.298243403350090
      | 
      |    1.374639155029902
      | 
      |    1.341605067579279
      | 
      |    1.252746560250751
      | 
      |    1.018313955486625
      | 
      |    0.129528294280125
      | 
      |    1.513997027979828
      | 
      |    1.387869811596475
      | 
      |    1.256061734211356
      | 
      |    0.990903629348201
      | 
      |    0.077920389236865
      | 
      |    1.200889162533513
      | 
      |    1.282379583523997
      | 
      |    1.565408012607870
      | 
      |    1.644736063700967
      | 
      |    1.534669709831138
      | 
      |    1.197888366617614
      | 
      |    1.286433748846038
      | 
      |    1.548840723589424
      | 
      |    1.925767481224847
      | 
      |    1.393369274193246
      | 
      |    0.955430677904952
      | 
      |    1.308685689453173
      | 
      |    1.610171776919144
      | 
      |    1.499862309464815
      | 
      |    1.265761278060954
      | 
      |    0.996265505273061
      | 
      |    1.429985826648748
      | 
      |    1.672233017060590
      | 
      |    1.347305108910380
      | 
      |    1.180924767286065
      | 
      |    1.153624069894655
      | 
      |    1.585076742513865
      | 
      |    1.603531375307336
      | 
      |    1.246765774696571
      | 
      |    1.150477028958167
      | 
      |    1.078522470990015
      | 
      |    1.144746261540051
      | 
      |    1.314678934955108
      | 
      |    1.599944308512642
      | 
      |    1.796913121984718
      | 
      |    1.088194694883578
      | 
      |    1.136583810467087
      | 
      |    1.322832623472215
      | 
      |    1.601423327990465
      | 
      |    1.783088655299468
      | 
      |    1.030599307373596
      | 
      |    1.041767602097911
      | 
      |    1.355912155063761
      | 
      |    1.574173111249969
      | 
      |    1.773134361038468
      | 
      |    0.777037927532027
      | 
      |    1.162391927866286
      | 
      |    1.359041122680662
      | 
      |    1.587110277582138
      | 
      |    1.816071161960944
      | 
      |    0.664684393667731
      | 
      |    1.336482260126401
      | 
      |    1.503551109181531
      | 
      |    1.246350986326241
      | 
      |    1.175931510283474
      | 
      |    1.219924206408560
      | 
      |    1.141847309137032
      | 
      |    1.347657081534498
      | 
      |    1.629730386754978
      | 
      |    1.723444332793390
      | 
      |    0.107048004021027
      | 
      |    1.151530005839755
      | 
      |    1.291470784284077
      | 
      |    1.549822039790982
      | 
      |    1.725321485032129
      | 
      |    1.146371080730706
      | 
      |    1.072833309536637
      | 
      |    1.297912796178577
      | 
      |    1.531920872426767
      | 
      |    1.698800516647542
      | 
      |    0.070449098384138
      | 
      |    1.121575424265131
      | 
      |    1.344641642506400
      | 
      |    1.527770314697527
      | 
      |    1.717465333395748
      | 
      |    0.584540283975742
      | 
      |    1.153865938787718
      | 
      |    1.396437575780084
      | 
      |    1.338134558357083
      | 
      |    1.203963950808773], [4 5 5])
  D Coeff Lookup : Lookup_n-D  NumberOfTableDimensions=3  BreakpointsForDimension1=[8 10 12 14]  BreakpointsForDimension2=[0 1 2 3 4]  BreakpointsForDimension3=[50 100 150 200 250]  Table=|  ExtrapMethod=Clip  UseLastTableValue=on  InternalRulePriority=Speed  RndMeth=Simplest  InputSameDT=on
      | reshape([     5.996127849086101e+02
      | 
      |      1.194264692275639e+03
      | 
      |      1.755311534748420e+03
      | 
      |      2.275962241291811e+03
      | 
      |      2.545703983297313e+03
      | 
      |      6.017336151931060e+02
      | 
      |      1.187808402100751e+03
      | 
      |      1.721769561030721e+03
      | 
      |      2.195180309800300e+03
      | 
      |      4.344113888159953e+03
      | 
      |      5.615361100914946e+02
      | 
      |      1.154418523048951e+03
      | 
      |      1.648435584451104e+03
      | 
      |      2.179797373831461e+03
      | 
      |      6.367939668589362e+03
      | 
      |      5.586800347742765e+02
      | 
      |      1.140498191262963e+03
      | 
      |      1.657475470600744e+03
      | 
      |      2.190163782172358e+03
      | 
      |      1.424668396564147e+04
      | 
      |      5.213468405795062e+02
      | 
      |      1.097756709721898e+03
      | 
      |      1.592704849377585e+03
      | 
      |      2.152124319372915e+03
      | 
      |      2.332116714432538e+04
      | 
      |      5.669081625318921e+02
      | 
      |      1.145341811867034e+03
      | 
      |      1.678064731477581e+03
      | 
      |      2.207574676784452e+03
      | 
      |      2.610491756678421e+03
      | 
      |      5.731297027478821e+02
      | 
      |      1.132486345612842e+03
      | 
      |      1.654089577735330e+03
      | 
      |      2.135900459060287e+03
      | 
      |      2.582007742139347e+03
      | 
      |      5.864970523461988e+02
      | 
      |      1.098395079765058e+03
      | 
      |      1.606837628755405e+03
      | 
      |      2.090772861419820e+03
      | 
      |      2.553936496604394e+03
      | 
      |      5.628146322511150e+02
      | 
      |      1.058917155196084e+03
      | 
      |      1.572437282696642e+03
      | 
      |      2.046072756070177e+03
      | 
      |      2.522700917363369e+03
      | 
      |      5.170520699440219e+02
      | 
      |      1.001140342755233e+03
      | 
      |      1.513799427865374e+03
      | 
      |      1.988675426585572e+03
      | 
      |      2.452473706672171e+03
      | 
      |      5.731871203055848e+02
      | 
      |      1.132588930886316e+03
      | 
      |      1.641130411306095e+03
      | 
      |      2.139432354773627e+03
      | 
      |      2.577568039021091e+03
      | 
      |      5.680952444433874e+02
      | 
      |      1.146653174842560e+03
      | 
      |      1.628864037881644e+03
      | 
      |      2.078585784530008e+03
      | 
      |      2.545198330421724e+03
      | 
      |      5.681071376317932e+02
      | 
      |      1.133067418581144e+03
      | 
      |      1.593676882089995e+03
      | 
      |      2.049036215361084e+03
      | 
      |      2.516128221959463e+03
      | 
      |      6.386772750709156e+02
      | 
      |      1.080428035490009e+03
      | 
      |      1.559613697974720e+03
      | 
      |      2.019575829634925e+03
      | 
      |      2.478847644542992e+03
      | 
      |      6.681324491028066e+02
      | 
      |      9.994349537610992e+02
      | 
      |      1.506043544146253e+03
      | 
      |      1.951902325832432e+03
      | 
      |      2.432670710119809e+03
      | 
      |      5.696088441080576e+02
      | 
      |      1.097297796317921e+03
      | 
      |      1.591537505834256e+03
      | 
      |      2.089522006613605e+03
      | 
      |      2.483202897646518e+03
      | 
      |      6.293016625928232e+03
      | 
      |      1.111172910222698e+03
      | 
      |      1.599511225258068e+03
      | 
      |      2.033720221818377e+03
      | 
      |      2.479403805121946e+03
      | 
      |      5.362026697911508e+02
      | 
      |      1.094903507948287e+03
      | 
      |      1.543037335368469e+03
      | 
      |      1.981067795316298e+03
      | 
      |      2.430497069020993e+03
      | 
      |      8.400779158467161e+03
      | 
      |      1.084090919418214e+03
      | 
      |      1.541286072134185e+03
      | 
      |      1.965337892878829e+03
      | 
      |      2.396313723125683e+03
      | 
      |      7.287937244164536e+02
      | 
      |      1.035449587490520e+03
      | 
      |      1.496128625234371e+03
      | 
      |      1.914361254730758e+03
      | 
      |      2.372998341607013e+03], [4 5 5])
  E Coeff Lookup : Lookup_n-D  NumberOfTableDimensions=3  BreakpointsForDimension1=[8 10 12 14]  BreakpointsForDimension2=[0 1 2 3 4]  BreakpointsForDimension3=[50 100 150 200 250]  Table=|  ExtrapMethod=Clip  UseLastTableValue=on  InternalRulePriority=Speed  RndMeth=Simplest  InputSameDT=on
      | reshape([   0.581170240520020
      | 
      |    0.513302065906332
      | 
      |   -0.110256215412594
      | 
      |   -0.841871678647663
      | 
      |    0.463315646533225
      | 
      |    0.549547356575374
      | 
      |    0.687620613348920
      | 
      |   -0.246060371305471
      | 
      |   -1.045560626592649
      | 
      |   -1.313853977136325
      | 
      |    0.511667156295047
      | 
      |    0.526457055135907
      | 
      |   -0.565837873518807
      | 
      |   -1.663813243957053
      | 
      |   -1.504115785530702
      | 
      |    0.481334683738741
      | 
      |   -0.251353231285475
      | 
      |   -0.886990791979627
      | 
      |   -1.768500017074065
      | 
      |   -1.460926069325169
      | 
      |    0.460776224478570
      | 
      |   -0.355178858750343
      | 
      |   -1.179864868777978
      | 
      |   -2.029253031595145
      | 
      |   -1.613653632705542
      | 
      |    0.530765335691638
      | 
      |    0.477789439547461
      | 
      |    0.429468797208466
      | 
      |    0.161716453575440
      | 
      |   -0.194411721664034
      | 
      |    0.517753487553597
      | 
      |    0.464393338378359
      | 
      |    0.446914135949458
      | 
      |    0.648053571992908
      | 
      |   -0.566128057660842
      | 
      |    0.371904289824661
      | 
      |    0.448548148271780
      | 
      |    0.443943060496705
      | 
      |   -0.032598282937631
      | 
      |   -1.007777334209280
      | 
      |    0.363814978823090
      | 
      |    0.456912839876029
      | 
      |    0.466283050108330
      | 
      |   -0.479334043993962
      | 
      |   -1.289027813894899
      | 
      |    0.409984852089051
      | 
      |    0.439162939101386
      | 
      |    0.236439669497680
      | 
      |   -0.998080152515394
      | 
      |   -1.535182350299851
      | 
      |    0.471551291603570
      | 
      |    0.426588322359852
      | 
      |    0.420720014282820
      | 
      |    0.399981871099958
      | 
      |    0.381966742060439
      | 
      |    0.434928184571716
      | 
      |    0.413178519461430
      | 
      |    0.426973790056562
      | 
      |    0.426906528858831
      | 
      |    0.403148477589051
      | 
      |    0.388314766661404
      | 
      |    0.360890343883042
      | 
      |    0.425263980508937
      | 
      |    0.422846670365782
      | 
      |    0.453978960977207
      | 
      |    0.239012560996651
      | 
      |    0.389900804698704
      | 
      |    0.426980263645195
      | 
      |    0.477306035174388
      | 
      |    0.603296856224376
      | 
      |    0.193377935782053
      | 
      |    0.421810808309948
      | 
      |    0.451847574903600
      | 
      |   -0.381275648156619
      | 
      |   -0.815723299506516
      | 
      |    0.513724699959696
      | 
      |    0.409551839124633
      | 
      |    0.435725112045746
      | 
      |    0.414873057215044
      | 
      |    0.390128460181774
      | 
      |    1.085743982874603
      | 
      |    0.405682012556922
      | 
      |    0.431385385577157
      | 
      |    0.431761097357240
      | 
      |    0.411449066150625
      | 
      |    0.389923720729443
      | 
      |    0.346014690155927
      | 
      |    0.417450436669446
      | 
      |    0.439809833241543
      | 
      |    0.442083898273286
      | 
      |    1.030462101038803
      | 
      |    0.372524919502987
      | 
      |    0.417500181663215
      | 
      |    0.444472612357413
      | 
      |    0.525246436100688
      | 
      |    0.156518406666601
      | 
      |    0.374213998985038
      | 
      |    0.451562356054846
      | 
      |    0.022834915270023
      | 
      |   -0.610936994003397], [4 5 5])
  B : Outport
  C : Outport  Port=2
  D : Outport  Port=3
  E : Outport  Port=4
  wires:
  Pressure/1 -> B Coeff Lookup/1, C Coeff Lookup/1, D Coeff Lookup/1, E Coeff Lookup/1
  Camber/1 -> B Coeff Lookup/2, E Coeff Lookup/2, D Coeff Lookup/2, C Coeff Lookup/2
  Normal Force/1 -> B Coeff Lookup/3, C Coeff Lookup/3, D Coeff Lookup/3, E Coeff Lookup/3
  B Coeff Lookup/1 -> B/1
  C Coeff Lookup/1 -> C/1
  D Coeff Lookup/1 -> D/1
  E Coeff Lookup/1 -> E/1

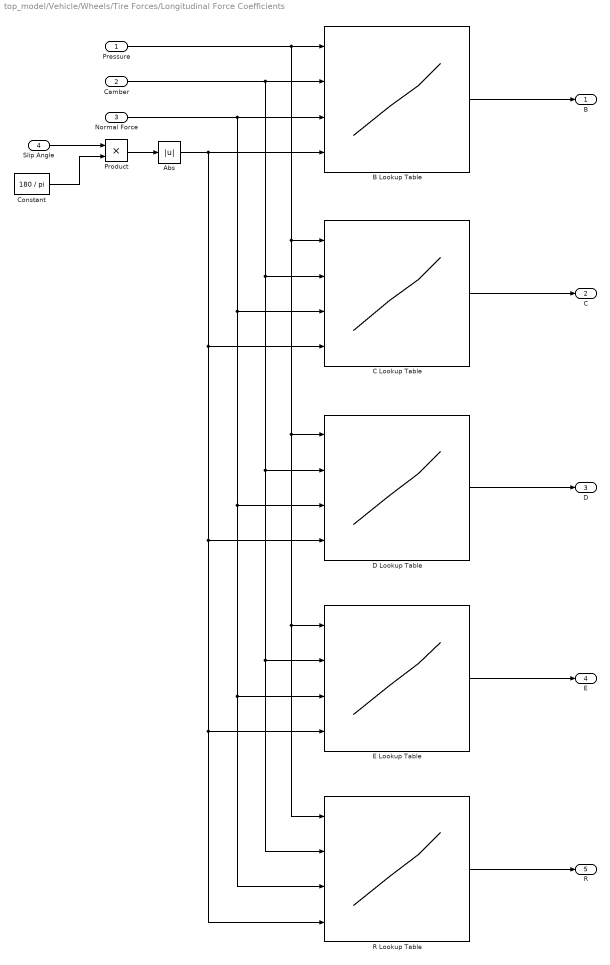
== system top_model/Vehicle/Wheels/Tire Forces/Longitudinal Force Coefficients ==
  Pressure : Inport
  Camber : Inport  Port=2
  Normal Force : Inport  Port=3
  Slip Angle : Inport  Port=4
  Abs : Abs
  B Lookup Table : Lookup_n-D  NumberOfTableDimensions=4  BreakpointsForDimension1=P  BreakpointsForDimension2=CA  BreakpointsForDimension3=F  BreakpointsForDimension4=S  Table=B  UseLastTableValue=on  InternalRulePriority=Speed  RndMeth=Simplest  InputSameDT=on
  C Lookup Table : Lookup_n-D  NumberOfTableDimensions=4  BreakpointsForDimension1=P  BreakpointsForDimension2=CA  BreakpointsForDimension3=F  BreakpointsForDimension4=S  Table=C  UseLastTableValue=on  InternalRulePriority=Speed  RndMeth=Simplest  InputSameDT=on
  Constant : Constant  Value=180 / pi
  D Lookup Table : Lookup_n-D  NumberOfTableDimensions=4  BreakpointsForDimension1=P  BreakpointsForDimension2=CA  BreakpointsForDimension3=F  BreakpointsForDimension4=S  Table=D  UseLastTableValue=on  InternalRulePriority=Speed  RndMeth=Simplest  InputSameDT=on
  E Lookup Table : Lookup_n-D  NumberOfTableDimensions=4  BreakpointsForDimension1=P  BreakpointsForDimension2=CA  BreakpointsForDimension3=F  BreakpointsForDimension4=S  Table=E  UseLastTableValue=on  InternalRulePriority=Speed  RndMeth=Simplest  InputSameDT=on
  Product : Product
  R Lookup Table : Lookup_n-D  NumberOfTableDimensions=4  BreakpointsForDimension1=P  BreakpointsForDimension2=CA  BreakpointsForDimension3=F  BreakpointsForDimension4=S  Table=R  ExtrapMethod=Clip  UseLastTableValue=on  InternalRulePriority=Speed  RndMeth=Simplest  InputSameDT=on
  B : Outport
  C : Outport  Port=2
  D : Outport  Port=3
  E : Outport  Port=4
  R : Outport  Port=5
  wires:
  Pressure/1 -> D Lookup Table/1, R Lookup Table/1, E Lookup Table/1, C Lookup Table/1, B Lookup Table/1
  Normal Force/1 -> C Lookup Table/3, D Lookup Table/3, R Lookup Table/3, E Lookup Table/3, B Lookup Table/3
  Abs/1 -> C Lookup Table/4, D Lookup Table/4, R Lookup Table/4, E Lookup Table/4, B Lookup Table/4
  B Lookup Table/1 -> B/1
  C Lookup Table/1 -> C/1
  D Lookup Table/1 -> D/1
  E Lookup Table/1 -> E/1
  Camber/1 -> C Lookup Table/2, D Lookup Table/2, R Lookup Table/2, E Lookup Table/2, B Lookup Table/2
  R Lookup Table/1 -> R/1
  Slip Angle/1 -> Product/1
  Constant/1 -> Product/2
  Product/1 -> Abs/1
